simulink model "Adaptive_Beamforming_ESC"  (R2026a)
settings: Solver=FixedStepDiscrete  StopTime=sim_time  FixedStep=sample_time
undefined symbols (not defined in the file): a_phi, a_theta, dspblkCoreblockFVToolHelper, gcbh, k_phi, k_theta, magnitude, omega_phi, omega_theta, physconst, sample_time, Thresh_Acq, Thresh_Drop
libraries: phasedtxrxlib x1, phasedbflib x1
settings Model: Creator=swaja  LastModifiedBy=swaja

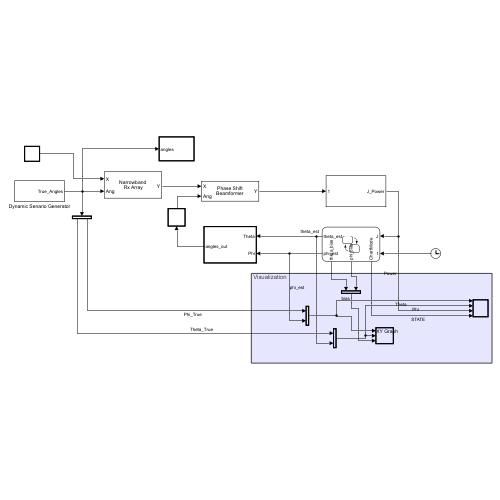
[thumbnail: Simulink's stored preview of the top-level diagram]
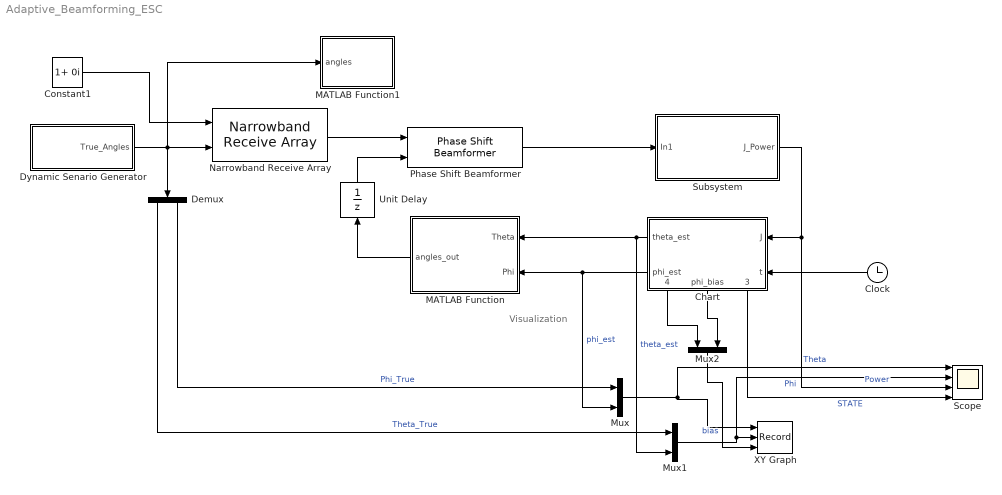
== system Adaptive_Beamforming_ESC ==
  note: Visualization
  Chart : Stateflow chart  TreatAsAtomicUnit=on
      settings: PortSchema="{\"entries\":[{\"content\":{\"sides\":[{\"content\":{\"connectorIds\":[\"Out1\",\"Out2\"]},\"type\":\"ConnectorPlacement.EquallySpacedRectSide\",\"uuid\":\"42747ea4-a3dc-464d-a499-c5e326f98ea9\"},{\"content\":{\"connectorIds\":[\"In1\",\"In2\"],\"side\":\"RIGHT\"},\"type\":\"ConnectorPlacement.EquallySpacedRectSide\",\"uuid\":\"689f8a55-f1e7-4e46-b33b-af78b9f0f391\"},{\"content\":{\"side\":\"TOP\"},\"type\":\"ConnectorPlacement.EquallySpacedRectSide\",\"uuid\":\"0df34723-e507-4cbd-9686-2346948b96cb\"},{\"content\":{\"connectorIds\":[\"Out4\",\"Out5\",\"Out3\"],\"side\":\"BOTTOM\"},\"type\":\"ConnectorPlacement.EquallySpacedRectSide\",\"uuid\":\"5a310151-0ba0-4c05-bb84-7781302f8bfa\"}]},\"type\":\"ConnectorPlacement.EquallySpacedConnector\",\"uuid\":\"d770fb89-b366-4c87-affa-cece0439bec1\"}],\"packageUris\":[\"http://schema.mathworks.com/mf0/Connector/R2020b\"],\"version\":\"1.0\"}"
  Clock : Clock
  Constant1 : Constant  Value=1+ 0i  OutDataTypeStr=double  SampleTime=sample_time
  Demux : Demux  Outputs=2
  Dynamic Senario Generator : Subsystem
  MATLAB Function : MATLAB Function  TreatAsAtomicUnit=on
  MATLAB Function1 : MATLAB Function  TreatAsAtomicUnit=on
  Mux : Mux  Inputs=2
  Mux1 : Mux  Inputs=2
  Mux2 : Mux  Inputs=2
  Narrowband Receive Array : phasedtxrxlib/Narrowband Receive Array  PropagationSpeed=physconst( 'LightSpeed' )  OperatingFrequency=fc  Wavefront=Plane  SensorGainMeasure=dB  Polarization=None  WeightsInputPort=off  SimulateUsing=Interpreted execution  Sensor=phased.URA(Size=[ M, N ],ElementSpacing=[ dx, dy ],Element=phased.IsotropicAntennaElement(FrequencyRange=freq_range))
  Phase Shift Beamformer : phasedbflib/Phase Shift Beamformer  PropagationSpeed=physconst( 'LightSpeed' )  OperatingFrequency=fc  DirectionSource=Input port  Direction=[ 0; 0 ]  NumPhaseShifterBits=0  WeightsNormalization=Distortionless  WeightsOutputPort=off  SimulateUsing=Interpreted execution  SensorArray=phased.URA(Size=[ M, N ],Element=phased.IsotropicAntennaElement(FrequencyRange=freq_range),ElementSpacing=[ dx, dy ])
  Scope : Scope  NumInputPorts=4
      settings: ActiveDisplayYMinimum=-56.25  ActiveDisplayYMaximum=56.25
  Subsystem : Subsystem
  Unit Delay : UnitDelay  SampleTime=-1
  XY Graph : Record  NumPorts=3.0  FileSettingsInternal="{\"entries\":[{\"content\":{\"excelSettings\":{\"content\":{},\"type\":\"Streamout.ExcelSettings\"},\"parquetSettings\":{\"content\":{},\"type\":\"Streamout.ParquetSettings\"}},\"type\":\"Streamout.FileSettingStorage\",\"uuid\":\"\"}],\"packageUris\":[\"http:\\/\\/schema.mathworks.com\\/mf0\\/streamout_blocks\\/R2020a\"],\"version\":\"1.0\"}"  FrameSettings=[0, 0, 0]  Layout=[1 1]  SignalsInternal="{\"entries\":[{\"content\":{\"signals\":[{\"content\":{\"blockPath\":[],\"dimensions\":[2],\"domain\":\"\",\"hasChildren\":true,\"lineColor\":\"#b746ff\",\"lineWidth\":2,\"port\":1,\"signalID\":1,\"signalName\":\"Theta\"},\"type\":\"RecordBlkView.Signal\",\"uuid\":\"\"},{\"content\":{\"blockPath\":[],\"channel\":[1],\"dimensions\":[2],\"domain\":\"\",\"lineColor\":\"#edb120\",\"lineWidth\":2,\"parentID\":1,\"plots\":[ 1 ],\"port\":1,\"signalID\":2,\"signalName\":\"Theta\"},\"type\":\"RecordBlkView.Signal\",\"uuid\":\"\"},{\"content\":{\"blockPath\":[],\"channel\":[2],\"dimensions\":[2],\"domain\":\"\",\"lineColor\":\"#139fff\",\"lineWidth\":2,\"parentID\":1,\"plots\":[ 1 ],\"port\":1,\"signalID\":3,\"signalName\":\"Theta\"},\"type\":\"RecordBlkView.Signal\",\"uuid\":\"\"},{\"content\":{\"blockPath\":[],\"dimensions\":[2],\"domain\":\"\",\"hasChildren\":true,\"lineColor\":\"#ff13a6\",\"lineWidth\":2,\"port\":2,\"signalID\":4,\"signalName\":\"Phi\"},\"type\":\"RecordBlkView.Signal\",\"uuid\":\"\"},{\"content\":{\"blockPath\":[],\"channel\":[1],\"dimensions\":[2],\"domain\":\"\",\"lineColor\":\"#edb120\",\"lineWidth\":2,\"parentID\":4,\"plots\":[ 1 ],\"port\":2,\"signalID\":5,\"signalName\":\"Phi\"},\"type\":\"RecordBlkView.Signal\",\"uuid\":\"\"},{\"content\":{\"blockPath\":[],\"channel\":[2],\"dimensions\":[2],\"domain\":\"\",\"lineColor\":\"#139fff\",\"lineWidth\":2,\"parentID\":4,\"plots\":[ 1 ],\"port\":2,\"signalID\":6,\"signalName\":\"Phi\"},\"type\":\"RecordBlkView.Signal\",\"uuid\":\"\"},{\"content\":{\"blockPath\":[],\"dimensions\":[2],\"domain\":\"\",\"hasChildren\":true,\"lineColor\":\"#22b573\",\"lineWidth\":2,\"port\":3,\"signalID\":7,\"signalName\":\"bias\"},\"type\":\"RecordBlkView.Signal\",\"uuid\":\"\"},{\"content\":{\"blockPath\":[],\"channel\":[1],\"dimensions\":[2],\"domain\":\"\",\"lineColor\":\"#b746ff\",\"lineWidth\":2,\"parentID\":7,\"plots\":[ 1 ],\"port\":3,\"signalID\":8,\"signalName\":\"bias\"},\"type\":\"RecordBlkView.Signal\",\"uuid\":\"\"},{\"content\":{\"blockPath\":[],\"channel\":[2],\"dimensions\":[2],\"domain\":\"\",\"lineColor\":\"#b746ff\",\"lineWidth\":2,\"parentID\":7,\"plots\":[ 1 ],\"port\":3,\"signalID\":9,\"signalName\":\"bias\"},\"type\":\"RecordBlkView.Signal\",\"uuid\":\"\"}]},\"type\":\"RecordBlkView.InputSignals\",\"uuid\":\"\"}],\"packageUris\":[\"http:\\/\\/schema.mathworks.com\\/mf0\\/streamout_blocks\\/R2020a\"],\"version\":\"1.0\"}"  VisualizationBindings="{\"xyplotplugin\":{\"info\":[{\"series\":[{\"bindingParametersList\":[{\"parameter\":\"X-Axis\",\"signalID\":3,\"signalName\":\"Theta(2)\"},{\"parameter\":\"Y-Axis\",\"signalID\":6,\"signalName\":\"Phi(2)\"}],\"seriesID\":0},{\"bindingParametersList\":[{\"parameter\":\"X-Axis\",\"signalID\":9,\"signalName\":\"bias(2)\"},{\"parameter\":\"Y-Axis\",\"signalID\":8,\"signalName\":\"bias(1)\"}],\"seriesID\":1},{\"bindingParametersList\":[{\"parameter\":\"X-Axis\",\"signalID\":2,\"signalName\":\"Theta(1)\"},{\"parameter\":\"Y-Axis\",\"signalID\":5,\"signalName\":\"Phi(1)\"}],\"seriesID\":2},{\"bindingParametersList\":[{\"parameter\":\"X-Axis\",\"signalID\":5,\"signalName\":\"Phi(1)\"}],\"seriesID\":3},{\"bindingParametersList\":[{\"parameter\":\"X-Axis\",\"signalID\":9,\"signalName\":\"bias(2)\"},{\"parameter\":\"Y-Axis\",\"signalID\":6,\"signalName\":\"Phi(2)\"}],\"seriesID\":4}],\"subplotID\":1}]}}"  CompatibilityTag=XY
  wires:
  Narrowband Receive Array/1 -> Phase Shift Beamformer/1
  Constant1/1 -> Narrowband Receive Array/1
  Phase Shift Beamformer/1 -> Subsystem/1(In1)
  Subsystem/1(J_Power) -> Scope/3, Chart/1(J)  "Power"
  Dynamic Senario Generator/1(True_Angles) -> MATLAB Function1/1(angles), Demux/1, Narrowband Receive Array/2
  Clock/1 -> Chart/2(t)
  Chart/1(theta_est) -> MATLAB Function/1(Theta), Mux1/2  "theta_est"
  Chart/2(phi_est) -> Mux/2, MATLAB Function/2(Phi)  "phi_est"
  Unit Delay/1 -> Phase Shift Beamformer/2
  MATLAB Function/1(angles_out) -> Unit Delay/1
  Demux/1 -> Mux1/1  "Theta_True"
  Demux/2 -> Mux/1  "Phi_True"
  Mux1/1 -> XY Graph/2, Scope/2  "Phi"
  Chart/3(ChartMode) -> Scope/4  "STATE"
  Mux/1 -> XY Graph/1, Scope/1  "Theta"
  Mux2/1 -> XY Graph/3  "bias"
  Chart/4(theta_bias) -> Mux2/1
  Chart/5(phi_bias) -> Mux2/2

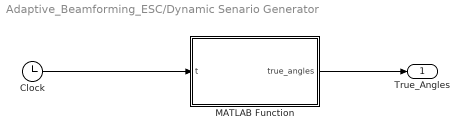
== system Adaptive_Beamforming_ESC/Dynamic Senario Generator ==
  Clock : Clock
  MATLAB Function : MATLAB Function  TreatAsAtomicUnit=on
  True_Angles : Outport
  wires:
  Clock/1 -> MATLAB Function/1(t)
  MATLAB Function/1(true_angles) -> True_Angles/1

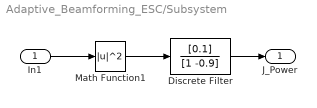
== system Adaptive_Beamforming_ESC/Subsystem ==
  In1 : Inport
  Discrete Filter : DiscreteFilter  LoadFcn=dspblkCoreblockFVToolHelper(gcbh,'load');  Numerator=[0.1]  Denominator=[1 -0.9]
      settings: CopyFcn=dspblkCoreblockFVToolHelper(gcbh,'copy');  DeleteFcn=dspblkCoreblockFVToolHelper(gcbh,'close');  ModelCloseFcn=dspblkCoreblockFVToolHelper(gcbh,'close');  PreSaveFcn=dspblkCoreblockFVToolHelper(gcbh,'presave');  PostSaveFcn=dspblkCoreblockFVToolHelper(gcbh,'postsave');  CloseFcn=dspblkCoreblockFVToolHelper(gcbh,'close');
  Math Function1 : Math  Operator=magnitude^2
  J_Power : Outport
  wires:
  Math Function1/1 -> Discrete Filter/1
  In1/1 -> Math Function1/1
  Discrete Filter/1 -> J_Power/1

== matlab function Adaptive_Beamforming_ESC/MATLAB Function ==
  data: Theta input; angles_out output; Phi input
function angles_out = packing(Theta, Phi)
    % This forces a strict 2x1 column vector: [Azimuth; Elevation]
    angles_out = [Theta; Phi];
end

== matlab function Adaptive_Beamforming_ESC/Dynamic Senario Generator/MATLAB Function ==
  data: t input; true_angles output
function true_angles = generate_trajectory(t)
    % Generate angles
    theta = 30 * sin(2 * pi * 0.1 * t); 
    phi = 10 * sin(2 * pi * 0.2 * t) + 10;

    % Force a strict 2x1 column vector
    true_angles = [theta; phi]; 
end

== stateflow chart Adaptive_Beamforming_ESC/Chart ==
  state INIT_SWEEP
    en:
    % Optional: Print to MATLAB command window to debug
    disp('Entering INIT_SWEEP: Searching for target...');
    du:
    % Fast scan covering a wide field of view
    theta_est = 45 * sin(2 * pi * 5 * t);
    phi_est = 20 * sin(2 * pi * 3 * t) + 10;
  state FINE_TRACKING
    en:
    disp('Target Locked: Executing ESC...');
    % Inherit the exact angle we found the signal at
    theta_bias = theta_est;
    phi_bias = phi_est;
    J_prev = J;
    du:
    % 1. High-Pass Filter
    HPF = J - J_prev;
    % 2. Demodulate to extract gradients
    grad_theta = HPF * sin(omega_theta * t);
    grad_phi = HPF * sin(omega_phi * t);
    % 3. Integrate to update biases
    theta_bias = theta_bias + (k_theta * grad_theta * sample_time);
    phi_bias = phi_bias + (k_phi * grad_phi * sample_time);
    % 4. Dither for physical outputs
    theta_est = theta_bias + a_theta * sin(omega_theta * t);
    phi_est = phi_bias + a_phi * sin(omega_phi * t);
    % 5. Store current power
    J_prev = J;
  state RECOVERY
    en:
    disp('Signal Lost: Attempting Recovery...');
    rec_time = 0; % Reset the recovery timer
    du:
    rec_time = rec_time + sample_time;
    % Expand the search dither by 3x, but keep the bias frozen
    theta_est = theta_bias + (a_theta * 3) * sin(omega_theta * t);
    phi_est = phi_bias + (a_phi * 3) * sin(omega_phi * t);
  (default) -> INIT_SWEEP
  INIT_SWEEP -> FINE_TRACKING : [J > Thresh_Acq]
  RECOVERY -> INIT_SWEEP [order 2] : [rec_time > 2.0]
  RECOVERY -> FINE_TRACKING [order 1] : [J > Thresh_Acq]
  FINE_TRACKING -> RECOVERY : [J < Thresh_Drop]
  data: J input; t input; theta_est output; phi_est output; J_prev local; a_phi parameter; Thresh_Acq parameter; Thresh_Drop parameter; a_theta parameter; k_phi parameter; k_theta parameter; omega_phi parameter; omega_theta parameter; sample_time parameter; HPF local; grad_phi local; grad_theta local; rec_time local; ChartMode output Enum: ChartModeType; theta_bias output; phi_bias output

== matlab function Adaptive_Beamforming_ESC/MATLAB Function1 ==
  data: angles input
function draw_beam(angles)
    % angles is your [theta; phi] vector coming from the ESC
    
    % coder.extrinsic allows Simulink to run standard MATLAB graphics functions
    coder.extrinsic('live_3D_beam');
    
    % Call our custom script and pass it the angles
    live_3D_beam(angles(1), angles(2));
end
